simulink model "JX_Kinect_multi_sync"  (Simulink 7.7)
settings: Solver=ode4  StartTime=0.0  StopTime=inf  FixedStep=sample_time  RelTol=1e-3
InitFcn:
  | sample_time=0.005;%0.004;%0.0025;%0.02;
  | DeltaT = 0.02;
  | g = 9.81;
  | H0 = g%0.3165;
  | Kl = 1;
  | 
  | Omega_r = 1.6;%for Horizontal reference
  | Zeta_r = 1; %for Horizontal reference
  | Omega = 1.8;%for Horizontal Control
  | Zeta = 0.5;    %for Horizontal Control
  | 
  | Omega_h_r = 2.5; %for vertical reference
  | Zeta_h_r = 0.8;  %for vertical reference
  | Omega_h = 2.7;    %for vertical control
  | Zeta_h = 0.8;         %for vertical control
  | PI=pi;
  | 
  | Mass = 1.15;
  | Acc_Max = 4;
  | Acc_Max_h = 4;
  | 
  | Max_RP = 60;
  | 
  | % for NN
  | n = 5;
  | r = 3;
  | n2 = 5;
  | NN_ST = 0.02;
  | 
  | GAMA_V = 6;
  | gama_V_e = 0.01;
  | 
  | GAMA_W = GAMA_V;
  | gama_W_e =0.01;
  | 
  | % deadzone
  | NN_Deadzone_Z = 0;
  | 
  | % inputs nomalizaton parameters
  | NN_Z_y_min = -3;
  | NN_Z_y_max = 0.5;
  | 
  | NN_Z_v_max = 8;
  | NN_Z_v_min = -NN_Z_v_max;
  | 
  | % alpha = 0.034;
  | alpha = 1;
  | % c_f = 0.0015;
  | c_f = 0.001;
  | c_y_tilt = 1*0.5;
  | 
  | %for WK paras
  | Heightcontrol = 0.08;
  | Scale_Factor=1;
  | yoffset=0;
  | 
  | load MaoBi_Oct04_2_int.mat
  | MB_Interp.time = [];
undefined symbols (not defined in the file or in its folder): DiscIntNeverNeededParam
libraries: simulink x15, X330_Control x6, dspadpt3 x6, nid_lib x2
(part 1 of 4)
settings Model: Creator=ttcl3  LastModifiedBy=Jx
settings SolverCC: MaxConsecutiveMinStep=auto
settings DebuggingCC: MultiTaskRateTransMsg=warning
settings SFSimCC: SimParseCustomCode=off

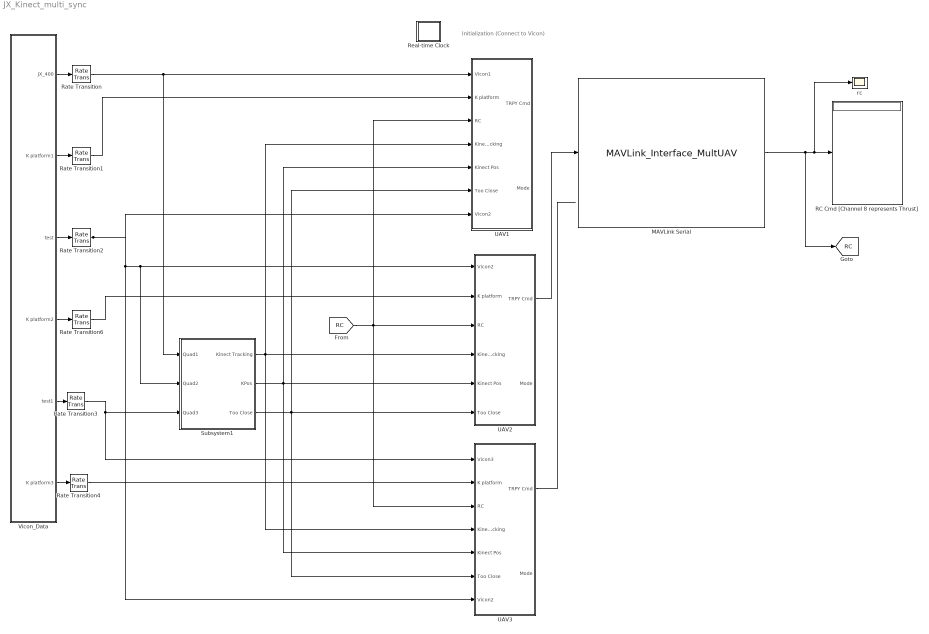
== system JX_Kinect_multi_sync ==
  note: Initialization
      | (Connect to Vicon)
  MAVLink Serial : S-Function  FunctionName=MAVLink_Interface_MultUAV  Parameters=COM_Port,Baud_Rate,MSG_INPUT,MSG_OUTPUT  EnableBusSupport=off  mask{COM_Port='COM6', Baud_Rate=57600, RC_SCALED=on, Quad_1=off, Quad_2=on, Quad_3=off}
      mask prompts: COM_Port "COM Port"; Baud_Rate "Baud Rate"; RC_SCALED "RC CHANNELS SCALED"; Quad_1 "Quad No 1"; Quad_2 "Quad No 2"; Quad_3 "Quad No 3"
      mask init:
      | MSG_ID_NUM_INPUT = [uint8(196) uint8(197) uint8(198)];
      | MSG_ID_NAME_INPUT = [Quad_1 Quad_2 Quad_3];
      | 
      | MSG_ID_NUM_OUTPUT = [uint8(34)];
      | MSG_ID_NAME_OUTPUT = [RC_SCALED];
      | 
      | idx_input = find(MSG_ID_NAME_INPUT);
      | MSG_INPUT = MSG_ID_NUM_INPUT(idx_input);
      | 
      | idx_output = find(MSG_ID_NAME_OUTPUT);
      | MSG_OUTPUT = MSG_ID_NUM_OUTPUT(idx_output);
      mask TabNameString: Setting,Setting,Output Message,Input Message,Input Message,Input Message
      mask Display:
      | % Block image
      | image(imread('10-inch Quad Heat Map.png'));
      | 
      | %Label block
      | fprintf('MAVLink Serial\n%s\n%dbps', COM_Port,  Baud_Rate)
      | 
      | 
      | %Label input ports
      | 
      | in = 1;
      | if (Quad_1 == 1)
      |     port_label('input', in, 'Quad 1');
      |     in = in + 1;
      | end
      | if (Quad_2 == 1)
      |     port_label('input', in, 'Quad 2');
      |     in = in + 1;
      | end
      | 
      | if (Quad_3 == 1)
      |     port_label('input', in, 'Quad 3');
      |     in = in + 1;
      | end
      | 
      | %Label output ports
      | 
      | out = 1;
      | if (RC_SCALED == 1)
      |     port_label('output', out, 'RC CMD');
      |     out = out + 1;
      | end
  RC Cmd [Channel 8 represents Thrust] : Display
  Rate Transition{,1..4,6} (6 alike) : RateTransition  OutPortSampleTime=0.02
  Real-time Clock : Subsystem  mask(Real-time Clock){sample_time=0.02, tolerance=1}
      mask prompts: sample_time "Synchronize with real-time every n seconds:"; tolerance "Real-time warning tolerance (seconds):"
      mask help: Real-time Synchronization Block
      mask Help: This block synchronizes simulation time with the PC real-time clock or UNIX system clock. The first dialog entry is the period at which the clock is checked to insure real-time synchronization. The second dialog entry is the number of seconds that the simulation time must be within real-time before a warning is printed.
      mask Display: plot(0,0,100,100,[40,60,60,54,54,64,69,76,82,77,81,83,83,81,78,74,70,64,57,49,41,35,32,30,30,31,34,40,47,47,40,40],[90,90,85,85,80,79,76,87,80,70,64,57,49,41,33,28,24,22,21,23,25,31,37,46,56,65,73,78,80,85,85,90],[69,53,53],[64,50,73])
  Subsystem1 : Subsystem
  UAV1 : Subsystem
  UAV2 : Subsystem
  UAV3 : Subsystem
  Vicon_Data : Subsystem
  rc : Scope
      settings: TimeRange=10  YMin=-1  YMax=0.1
  tag scope: RC=global
  wires:
  MAVLink Serial/1 -> [RC], RC Cmd [Channel 8 represents Thrust]/1, rc/1
  Vicon_Data/1(JX_400) -> Rate Transition/1
  Vicon_Data/2(K platform1) -> Rate Transition1/1
  Rate Transition/1 -> UAV1/1(Vicon1), Subsystem1/1(Quad1)
  Rate Transition1/1 -> UAV1/2(K platform)
  Vicon_Data/3(test) -> Rate Transition2/1
  Rate Transition2/1 -> UAV1/7(Vicon2), UAV3/7(Vicon2), UAV2/1(Vicon2), Subsystem1/2(Quad2)
  Vicon_Data/4(K platform2) -> Rate Transition6/1
  Vicon_Data/5(test1) -> Rate Transition3/1
  Rate Transition3/1 -> UAV3/1(Vicon3), Subsystem1/3(Quad3)
  UAV3/1(TRPY Cmd) -> ?
  Vicon_Data/6(K platform3) -> Rate Transition4/1
  Rate Transition4/1 -> UAV3/2(K platform)
  Rate Transition6/1 -> UAV2/2(K platform)
  [RC] -> UAV1/3(RC), UAV2/3(RC), UAV3/3(RC)
  Subsystem1/1(Kinect Tracking) -> UAV2/4(Kinect Tracking), UAV1/4(Kinect Tracking), UAV3/4(Kinect Tracking)
  Subsystem1/2(KPos) -> UAV2/5(Kinect Pos), UAV1/5(Kinect Pos), UAV3/5(Kinect Pos)
  Subsystem1/3(Too Close) -> UAV1/6(Too Close), UAV2/6(Too Close), UAV3/6(Too Close)
  UAV2/1(TRPY Cmd) -> MAVLink Serial/1

== system JX_Kinect_multi_sync/Real-time Clock ==
  Real-time Clock : S-Function  FunctionName=rtclock  Parameters=sample_time, tolerance  EnableBusSupport=off

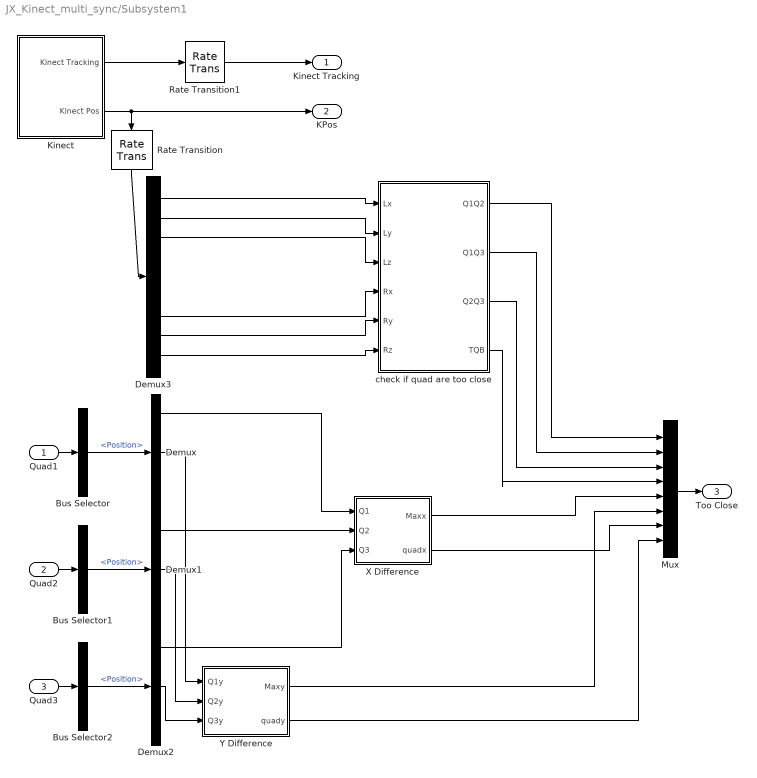
== system JX_Kinect_multi_sync/Subsystem1 ==
  Quad1 : Inport
  Quad2 : Inport  Port=2
  Quad3 : Inport  Port=3
  Bus Selector : BusSelector  OutputSignals=Position
  Bus Selector1 : BusSelector  OutputSignals=Position
  Bus Selector2 : BusSelector  OutputSignals=Position
  Demux : Demux  Outputs=3
  Demux1 : Demux  Outputs=3
  Demux2 : Demux  Outputs=3
  Demux3 : Demux  Outputs=9
  Kinect : Subsystem
  Mux : Mux  Inputs=8
  Rate Transition : RateTransition
  Rate Transition1 : RateTransition
  X Difference : Subsystem
  Y Difference : Subsystem
  check if quad are too close : Stateflow chart  TreatAsAtomicUnit=on
  Kinect Tracking : Outport
  KPos : Outport  Port=2
  Too Close : Outport  Port=3
  wires:
  Kinect/2(Kinect Pos) -> KPos/1, Rate Transition/1
  Kinect/1(Kinect Tracking) -> Rate Transition1/1
  Bus Selector/1 -> Demux/1  "<Position>"
  Bus Selector1/1 -> Demux1/1  "<Position>"
  Bus Selector2/1 -> Demux2/1  "<Position>"
  Quad2/1 -> Bus Selector1/1
  Quad3/1 -> Bus Selector2/1
  Quad1/1 -> Bus Selector/1
  Demux3/1 -> check if quad are too close/1(Lx)
  Demux3/2 -> check if quad are too close/2(Ly)
  Demux3/3 -> check if quad are too close/3(Lz)
  Demux3/7 -> check if quad are too close/4(Rx)
  Demux3/8 -> check if quad are too close/5(Ry)
  Demux3/9 -> check if quad are too close/6(Rz)
  Demux/1 -> X Difference/1(Q1)
  Demux/2 -> Y Difference/1(Q1y)
  Demux1/1 -> X Difference/2(Q2)
  Demux2/1 -> X Difference/3(Q3)
  check if quad are too close/1(Q1Q2) -> Mux/1
  check if quad are too close/2(Q1Q3) -> Mux/2
  check if quad are too close/3(Q2Q3) -> Mux/3
  Mux/1 -> Too Close/1
  check if quad are too close/4(TQB) -> Mux/4
  Y Difference/1(Maxy) -> Mux/6
  X Difference/1(Maxx) -> Mux/5
  X Difference/2(quadx) -> Mux/7
  Y Difference/2(quady) -> Mux/8
  Demux1/2 -> Y Difference/2(Q2y)
  Demux2/2 -> Y Difference/3(Q3y)
  Rate Transition/1 -> Demux3/1
  Rate Transition1/1 -> Kinect Tracking/1

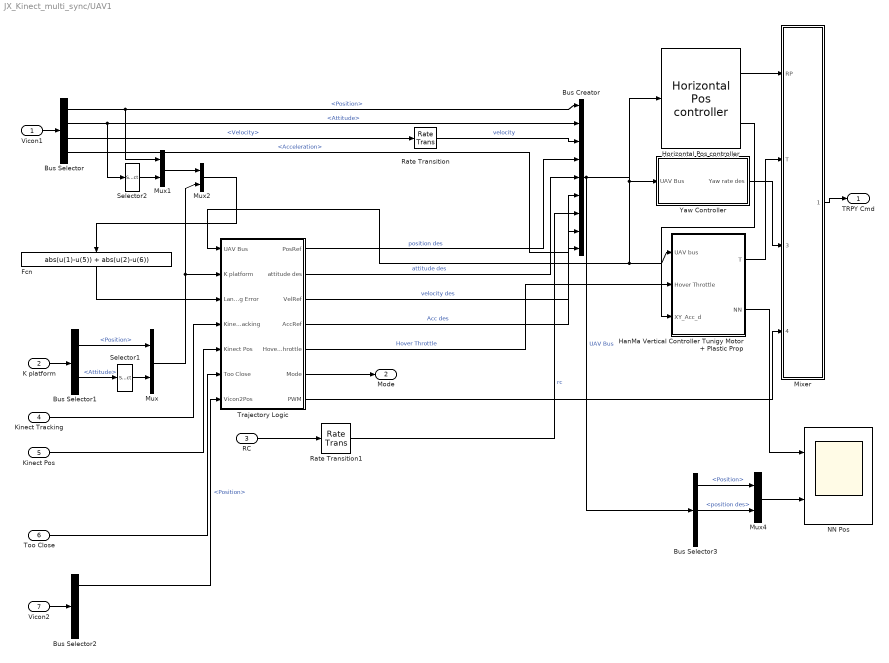
== system JX_Kinect_multi_sync/UAV1 ==
  Vicon1 : Inport
  K platform : Inport  Port=2
  RC : Inport  Port=3
  Kinect Tracking : Inport  Port=4
  Kinect Pos : Inport  Port=5
  Too Close : Inport  Port=6
  Vicon2 : Inport  Port=7
  Bus Creator : BusCreator  Inputs=9
  Bus Selector : BusSelector  OutputSignals=Position,Attitude,Velocity,Acceleration
  Bus Selector1 : BusSelector  OutputSignals=Position,Attitude
  Bus Selector2 : BusSelector  OutputSignals=Position,Attitude,Velocity,Acceleration
  Bus Selector3 : BusSelector  OutputSignals=Position,position des,Attitude
  Fcn : Fcn  Expr=abs(u(1)-u(5)) + abs(u(2)-u(6))
  HanMa Vertical Controller Tunigy Motor + Plastic Prop : Subsystem  mask{Omega_h=Omega_h, Zeta_h=Zeta_h, PID_I_h=0, mass=0.85}
      mask prompts: Omega_h "Omega (P Gain  = Omega^2)"; Zeta_h "Zeta (D Gain = 2*Omega*Zeta)"; PID_I_h "I Gain"
      mask TabNameString: Control Paramters,Control Paramters,Control Paramters,Mass
  Horizontal Pos controller : X330_Control/Horizontal Pos controller  SystemSampleTime=-1  Max_RP=Max_RP  Omega=Omega  PID_i=2  Zeta=Zeta
  Mixer : Subsystem
  Mux{,1..2,4} (4 alike) : Mux  Inputs=2
  NN Pos : Scope  NumInputPorts=2
      settings: TimeRange=90  YMin=-5~-2  YMax=10~2  SaveName=ScopeData3
  Rate Transition : RateTransition  OutPortSampleTime=0.02
  Rate Transition1 : RateTransition  OutPortSampleTime=0.02
  Selector1 : Selector  InputPortWidth=3  IndexOptions=Index vector (dialog)  Indices=[3]  OutputSizes=1
  Selector2 : Selector  InputPortWidth=3  IndexOptions=Index vector (dialog)  Indices=[3]  OutputSizes=1
  Trajectory Logic : Subsystem
  Yaw Controller : Subsystem
  TRPY Cmd : Outport
  Mode : Outport  Port=2
  wires:
  Horizontal Pos controller/1 -> Mixer/1(RP)
  Rate Transition/1 -> Bus Creator/3  "velocity"
  Rate Transition1/1 -> Bus Creator/7  "rc"
  Bus Creator/1 -> Yaw Controller/1(UAV Bus), Trajectory Logic/1(UAV Bus), HanMa Vertical Controller Tunigy Motor + Plastic Prop/1(UAV bus), Horizontal Pos controller/1, Bus Selector3/1  "UAV Bus"
  Yaw Controller/1(Yaw rate des) -> Mixer/3(Yaw rate)
  HanMa Vertical Controller Tunigy Motor + Plastic Prop/1(T) -> Mixer/2(T)
  Bus Selector/4 -> Bus Creator/8  "<Acceleration>"
  Trajectory Logic/1(PosRef) -> Bus Creator/4  "position des"
  Trajectory Logic/2(attitude des) -> Bus Creator/5  "attitude des"
  Trajectory Logic/3(VelRef) -> Bus Creator/6  "velocity des"
  Trajectory Logic/5(HoverThrottle) -> HanMa Vertical Controller Tunigy Motor + Plastic Prop/2(Hover Throttle)  "Hover Throttle"
  Bus Selector/1 -> Mux1/1, Bus Creator/1  "<Position>"
  Bus Selector/2 -> Selector2/1, Bus Creator/2  "<Attitude>"
  Bus Selector/3 -> Rate Transition/1  "<Velocity>"
  Vicon1/1 -> Bus Selector/1
  Mixer/1(XYZ RPY) -> TRPY Cmd/1
  Trajectory Logic/4(AccRef) -> Bus Creator/9  "Acc des"
  Mux/1 -> Mux2/2, Trajectory Logic/2(K platform)
  Trajectory Logic/6(Mode) -> Mode/1
  RC/1 -> Rate Transition1/1
  Trajectory Logic/7(PWM) -> Mixer/4(PWM)
  K platform/1 -> Bus Selector1/1
  Bus Selector1/1 -> Mux/1  "<Position>"
  Bus Selector1/2 -> Selector1/1  "<Attitude>"
  Selector1/1 -> Mux/2
  Selector2/1 -> Mux1/2
  Mux2/1 -> Fcn/1
  Mux1/1 -> Mux2/1
  Fcn/1 -> Trajectory Logic/3(Landing Error)
  Horizontal Pos controller/2 -> HanMa Vertical Controller Tunigy Motor + Plastic Prop/3(XY_Acc_d)
  Mux4/1 -> NN Pos/2
  Bus Selector3/1 -> Mux4/1  "<Position>"
  Bus Selector3/2 -> Mux4/2  "<position des>"
  HanMa Vertical Controller Tunigy Motor + Plastic Prop/2(NN) -> NN Pos/1
  Kinect Tracking/1 -> Trajectory Logic/4(Kinect Tracking)
  Kinect Pos/1 -> Trajectory Logic/5(Kinect Pos)
  Too Close/1 -> Trajectory Logic/6(Too Close)
  Vicon2/1 -> Bus Selector2/1
  Bus Selector2/1 -> Trajectory Logic/7(Vicon2Pos)  "<Position>"

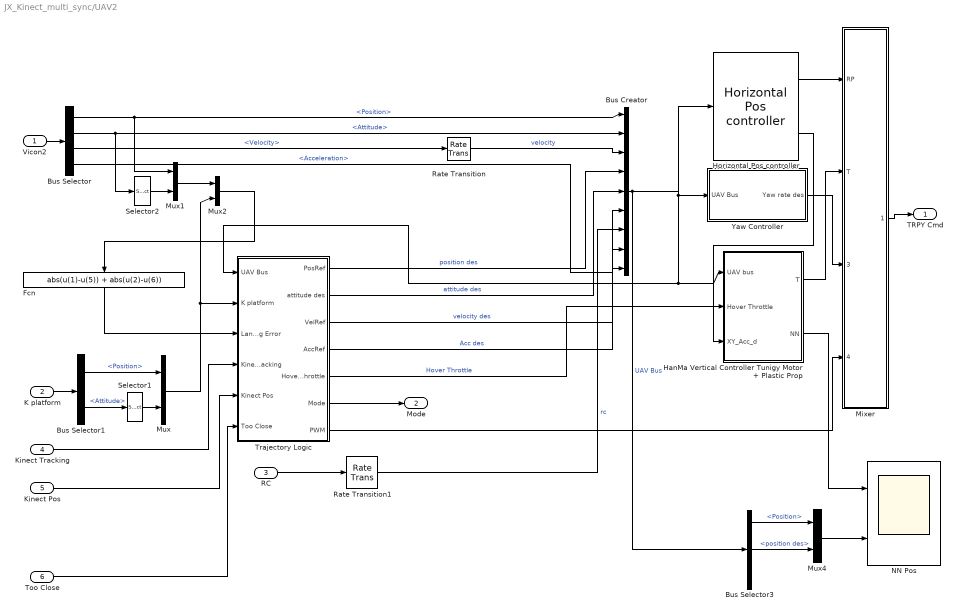
== system JX_Kinect_multi_sync/UAV2 ==
  Vicon2 : Inport
  K platform : Inport  Port=2
  RC : Inport  Port=3
  Kinect Tracking : Inport  Port=4
  Kinect Pos : Inport  Port=5
  Too Close : Inport  Port=6
  Bus Creator : BusCreator  Inputs=9
  Bus Selector : BusSelector  OutputSignals=Position,Attitude,Velocity,Acceleration
  Bus Selector1 : BusSelector  OutputSignals=Position,Attitude
  Bus Selector3 : BusSelector  OutputSignals=Position,position des,Attitude
  Fcn : Fcn  Expr=abs(u(1)-u(5)) + abs(u(2)-u(6))
  HanMa Vertical Controller Tunigy Motor + Plastic Prop : Subsystem  mask{Omega_h=Omega_h, Zeta_h=Zeta_h, PID_I_h=0, mass=0.85}
      mask prompts: Omega_h "Omega (P Gain  = Omega^2)"; Zeta_h "Zeta (D Gain = 2*Omega*Zeta)"; PID_I_h "I Gain"
      mask TabNameString: Control Paramters,Control Paramters,Control Paramters,Mass
  Horizontal Pos controller : X330_Control/Horizontal Pos controller  SystemSampleTime=-1  Max_RP=Max_RP  Omega=Omega  PID_i=2  Zeta=Zeta
  Mixer : Subsystem
  Mux{,1..2,4} (4 alike) : Mux  Inputs=2
  NN Pos : Scope  NumInputPorts=2
      settings: TimeRange=90  YMin=-5~-2  YMax=10~2  SaveName=ScopeData3
  Rate Transition : RateTransition  OutPortSampleTime=0.02
  Rate Transition1 : RateTransition  OutPortSampleTime=0.02
  Selector1 : Selector  InputPortWidth=3  IndexOptions=Index vector (dialog)  Indices=[3]  OutputSizes=1
  Selector2 : Selector  InputPortWidth=3  IndexOptions=Index vector (dialog)  Indices=[3]  OutputSizes=1
  Trajectory Logic : Subsystem
  Yaw Controller : Subsystem
  TRPY Cmd : Outport
  Mode : Outport  Port=2
  wires:
  Horizontal Pos controller/1 -> Mixer/1(RP)
  Rate Transition/1 -> Bus Creator/3  "velocity"
  Rate Transition1/1 -> Bus Creator/7  "rc"
  Bus Creator/1 -> Yaw Controller/1(UAV Bus), Trajectory Logic/1(UAV Bus), HanMa Vertical Controller Tunigy Motor + Plastic Prop/1(UAV bus), Horizontal Pos controller/1, Bus Selector3/1  "UAV Bus"
  Yaw Controller/1(Yaw rate des) -> Mixer/3(Yaw rate)
  HanMa Vertical Controller Tunigy Motor + Plastic Prop/1(T) -> Mixer/2(T)
  Bus Selector/4 -> Bus Creator/8  "<Acceleration>"
  Trajectory Logic/1(PosRef) -> Bus Creator/4  "position des"
  Trajectory Logic/2(attitude des) -> Bus Creator/5  "attitude des"
  Trajectory Logic/3(VelRef) -> Bus Creator/6  "velocity des"
  Trajectory Logic/5(HoverThrottle) -> HanMa Vertical Controller Tunigy Motor + Plastic Prop/2(Hover Throttle)  "Hover Throttle"
  Bus Selector/1 -> Mux1/1, Bus Creator/1  "<Position>"
  Bus Selector/2 -> Selector2/1, Bus Creator/2  "<Attitude>"
  Bus Selector/3 -> Rate Transition/1  "<Velocity>"
  Vicon2/1 -> Bus Selector/1
  Mixer/1(XYZ RPY) -> TRPY Cmd/1
  Trajectory Logic/4(AccRef) -> Bus Creator/9  "Acc des"
  Mux/1 -> Mux2/2, Trajectory Logic/2(K platform)
  Trajectory Logic/6(Mode) -> Mode/1
  RC/1 -> Rate Transition1/1
  Trajectory Logic/7(PWM) -> Mixer/4(PWM)
  K platform/1 -> Bus Selector1/1
  Bus Selector1/1 -> Mux/1  "<Position>"
  Bus Selector1/2 -> Selector1/1  "<Attitude>"
  Selector1/1 -> Mux/2
  Selector2/1 -> Mux1/2
  Mux2/1 -> Fcn/1
  Mux1/1 -> Mux2/1
  Fcn/1 -> Trajectory Logic/3(Landing Error)
  Horizontal Pos controller/2 -> HanMa Vertical Controller Tunigy Motor + Plastic Prop/3(XY_Acc_d)
  Mux4/1 -> NN Pos/2
  Bus Selector3/1 -> Mux4/1  "<Position>"
  Bus Selector3/2 -> Mux4/2  "<position des>"
  HanMa Vertical Controller Tunigy Motor + Plastic Prop/2(NN) -> NN Pos/1
  Kinect Tracking/1 -> Trajectory Logic/4(Kinect Tracking)
  Kinect Pos/1 -> Trajectory Logic/5(Kinect Pos)
  Too Close/1 -> Trajectory Logic/6(Too Close)

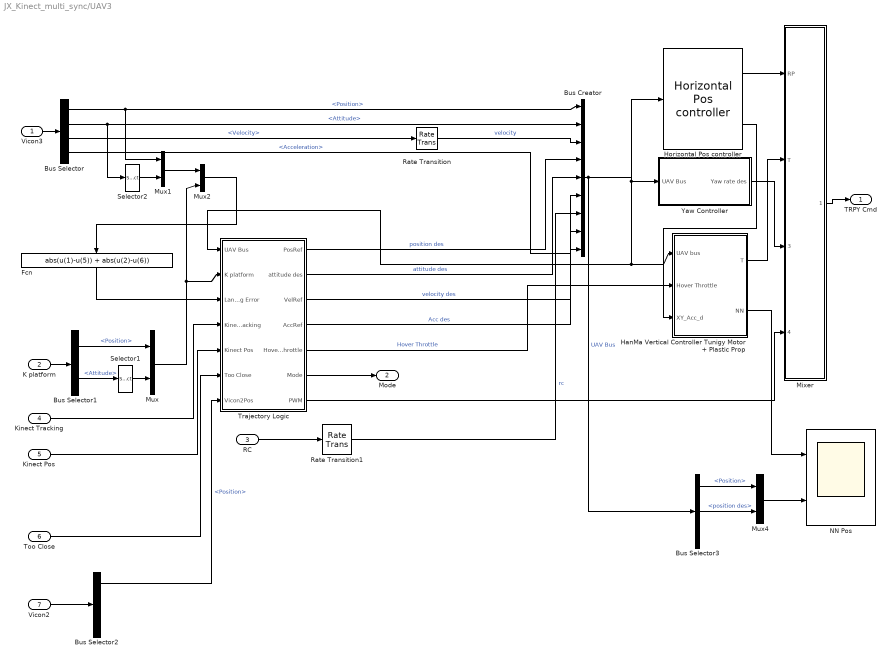
== system JX_Kinect_multi_sync/UAV3 ==
  Vicon3 : Inport
  K platform : Inport  Port=2
  RC : Inport  Port=3
  Kinect Tracking : Inport  Port=4
  Kinect Pos : Inport  Port=5
  Too Close : Inport  Port=6
  Vicon2 : Inport  Port=7
  Bus Creator : BusCreator  Inputs=9
  Bus Selector : BusSelector  OutputSignals=Position,Attitude,Velocity,Acceleration
  Bus Selector1 : BusSelector  OutputSignals=Position,Attitude
  Bus Selector2 : BusSelector  OutputSignals=Position,Attitude,Velocity,Acceleration
  Bus Selector3 : BusSelector  OutputSignals=Position,position des,Attitude
  Fcn : Fcn  Expr=abs(u(1)-u(5)) + abs(u(2)-u(6))
  HanMa Vertical Controller Tunigy Motor + Plastic Prop : Subsystem  mask{Omega_h=Omega_h, Zeta_h=Zeta_h, PID_I_h=0, mass=0.85}
      mask prompts: Omega_h "Omega (P Gain  = Omega^2)"; Zeta_h "Zeta (D Gain = 2*Omega*Zeta)"; PID_I_h "I Gain"
      mask TabNameString: Control Paramters,Control Paramters,Control Paramters,Mass
  Horizontal Pos controller : X330_Control/Horizontal Pos controller  SystemSampleTime=-1  Max_RP=Max_RP  Omega=Omega  PID_i=2  Zeta=Zeta
  Mixer : Subsystem
  Mux{,1..2,4} (4 alike) : Mux  Inputs=2
  NN Pos : Scope  NumInputPorts=2
      settings: TimeRange=90  YMin=-5~-2  YMax=10~2  SaveName=ScopeData3
  Rate Transition : RateTransition  OutPortSampleTime=0.02
  Rate Transition1 : RateTransition  OutPortSampleTime=0.02
  Selector1 : Selector  InputPortWidth=3  IndexOptions=Index vector (dialog)  Indices=[3]  OutputSizes=1
  Selector2 : Selector  InputPortWidth=3  IndexOptions=Index vector (dialog)  Indices=[3]  OutputSizes=1
  Trajectory Logic : Subsystem
  Yaw Controller : Subsystem
  TRPY Cmd : Outport
  Mode : Outport  Port=2
  wires:
  Horizontal Pos controller/1 -> Mixer/1(RP)
  Rate Transition/1 -> Bus Creator/3  "velocity"
  Rate Transition1/1 -> Bus Creator/7  "rc"
  Bus Creator/1 -> Yaw Controller/1(UAV Bus), Trajectory Logic/1(UAV Bus), HanMa Vertical Controller Tunigy Motor + Plastic Prop/1(UAV bus), Horizontal Pos controller/1, Bus Selector3/1  "UAV Bus"
  Yaw Controller/1(Yaw rate des) -> Mixer/3(Yaw rate)
  HanMa Vertical Controller Tunigy Motor + Plastic Prop/1(T) -> Mixer/2(T)
  Bus Selector/4 -> Bus Creator/8  "<Acceleration>"
  Trajectory Logic/1(PosRef) -> Bus Creator/4  "position des"
  Trajectory Logic/2(attitude des) -> Bus Creator/5  "attitude des"
  Trajectory Logic/3(VelRef) -> Bus Creator/6  "velocity des"
  Trajectory Logic/5(HoverThrottle) -> HanMa Vertical Controller Tunigy Motor + Plastic Prop/2(Hover Throttle)  "Hover Throttle"
  Bus Selector/1 -> Mux1/1, Bus Creator/1  "<Position>"
  Bus Selector/2 -> Selector2/1, Bus Creator/2  "<Attitude>"
  Bus Selector/3 -> Rate Transition/1  "<Velocity>"
  Vicon3/1 -> Bus Selector/1
  Mixer/1(XYZ RPY) -> TRPY Cmd/1
  Trajectory Logic/4(AccRef) -> Bus Creator/9  "Acc des"
  Mux/1 -> Mux2/2, Trajectory Logic/2(K platform)
  Trajectory Logic/6(Mode) -> Mode/1
  RC/1 -> Rate Transition1/1
  Trajectory Logic/7(PWM) -> Mixer/4(PWM)
  K platform/1 -> Bus Selector1/1
  Bus Selector1/1 -> Mux/1  "<Position>"
  Bus Selector1/2 -> Selector1/1  "<Attitude>"
  Selector1/1 -> Mux/2
  Selector2/1 -> Mux1/2
  Mux2/1 -> Fcn/1
  Mux1/1 -> Mux2/1
  Fcn/1 -> Trajectory Logic/3(Landing Error)
  Horizontal Pos controller/2 -> HanMa Vertical Controller Tunigy Motor + Plastic Prop/3(XY_Acc_d)
  Mux4/1 -> NN Pos/2
  Bus Selector3/1 -> Mux4/1  "<Position>"
  Bus Selector3/2 -> Mux4/2  "<position des>"
  HanMa Vertical Controller Tunigy Motor + Plastic Prop/2(NN) -> NN Pos/1
  Kinect Tracking/1 -> Trajectory Logic/4(Kinect Tracking)
  Kinect Pos/1 -> Trajectory Logic/5(Kinect Pos)
  Too Close/1 -> Trajectory Logic/6(Too Close)
  Vicon2/1 -> Bus Selector2/1
  Bus Selector2/1 -> Trajectory Logic/7(Vicon2Pos)  "<Position>"

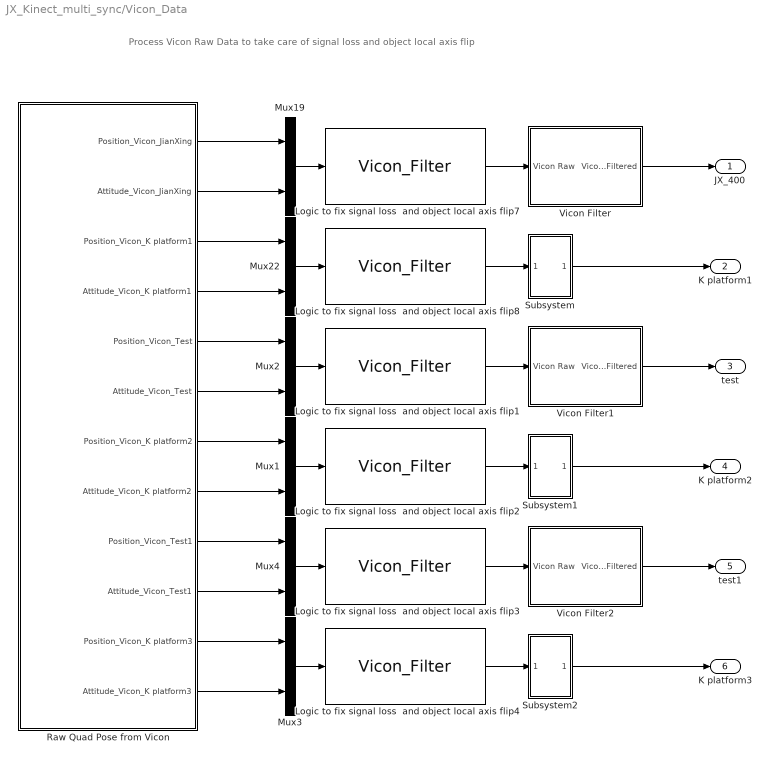
== system JX_Kinect_multi_sync/Vicon_Data ==
  note: Process Vicon Raw Data to take care of signal loss and object local axis flip
  Logic to fix signal loss  and object local axis flip{1..4,7..8} (6 alike) : M-S-Function  FunctionName=Vicon_Filter
  Mux{1..4,19,22} (6 alike) : Mux  Inputs=2
  Raw Quad Pose from Vicon : Subsystem
  Subsystem : Subsystem
  Subsystem1 : Subsystem
  Subsystem2 : Subsystem
  Vicon Filter : Subsystem
  Vicon Filter1 : Subsystem
  Vicon Filter2 : Subsystem
  JX_400 : Outport
  K platform1 : Outport  Port=2
  test : Outport  Port=3
  K platform2 : Outport  Port=4
  test1 : Outport  Port=5
  K platform3 : Outport  Port=6
  wires:
  Raw Quad Pose from Vicon/4(Attitude_Vicon_K platform1) -> Mux22/2
  Raw Quad Pose from Vicon/3(Position_Vicon_K platform1) -> Mux22/1
  Raw Quad Pose from Vicon/2(Attitude_Vicon_JianXing) -> Mux19/2
  Raw Quad Pose from Vicon/1(Position_Vicon_JianXing) -> Mux19/1
  Subsystem/1(Out1) -> K platform1/1
  Logic to fix signal loss  and object local axis flip8/1 -> Subsystem/1(In1)
  Mux22/1 -> Logic to fix signal loss  and object local axis flip8/1
  Vicon Filter/1(Vicon Filtered) -> JX_400/1
  Logic to fix signal loss  and object local axis flip7/1 -> Vicon Filter/1(Vicon Raw)
  Mux19/1 -> Logic to fix signal loss  and object local axis flip7/1
  Logic to fix signal loss  and object local axis flip1/1 -> Vicon Filter1/1(Vicon Raw)
  Vicon Filter1/1(Vicon Filtered) -> test/1
  Raw Quad Pose from Vicon/6(Attitude_Vicon_Test) -> Mux2/2
  Raw Quad Pose from Vicon/5(Position_Vicon_Test) -> Mux2/1
  Mux2/1 -> Logic to fix signal loss  and object local axis flip1/1
  Subsystem1/1(Out1) -> K platform2/1
  Logic to fix signal loss  and object local axis flip2/1 -> Subsystem1/1(In1)
  Mux1/1 -> Logic to fix signal loss  and object local axis flip2/1
  Raw Quad Pose from Vicon/7(Position_Vicon_K platform2) -> Mux1/1
  Raw Quad Pose from Vicon/8(Attitude_Vicon_K platform2) -> Mux1/2
  Logic to fix signal loss  and object local axis flip3/1 -> Vicon Filter2/1(Vicon Raw)
  Vicon Filter2/1(Vicon Filtered) -> test1/1
  Raw Quad Pose from Vicon/10(Attitude_Vicon_Test1) -> Mux4/2
  Raw Quad Pose from Vicon/9(Position_Vicon_Test1) -> Mux4/1
  Mux4/1 -> Logic to fix signal loss  and object local axis flip3/1
  Subsystem2/1(Out1) -> K platform3/1
  Logic to fix signal loss  and object local axis flip4/1 -> Subsystem2/1(In1)
  Mux3/1 -> Logic to fix signal loss  and object local axis flip4/1
  Raw Quad Pose from Vicon/11(Position_Vicon_K platform3) -> Mux3/1
  Raw Quad Pose from Vicon/12(Attitude_Vicon_K platform3) -> Mux3/2

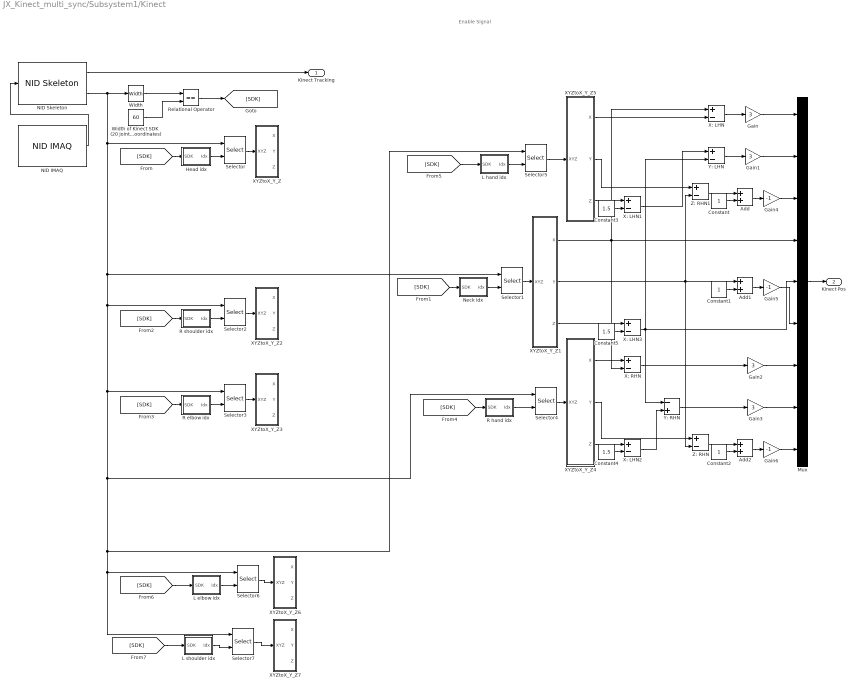
== system JX_Kinect_multi_sync/Subsystem1/Kinect ==
  note: Enable Signal
  Add : Sum
  Add1 : Sum
  Add2 : Sum
  Constant : Constant
  Constant1 : Constant
  Constant2 : Constant
  Constant3 : Constant  Value=1.5
  Constant4 : Constant  Value=1.5
  Constant5 : Constant  Value=1.5
  Gain{,1..3} (4 alike) : Gain  Gain=3
  Gain4 : Gain  Gain=-1
  Gain5 : Gain  Gain=-1
  Gain6 : Gain  Gain=-1
  Head idx : Subsystem
  L elbow idx : Subsystem
  L hand idx : Subsystem
  L shoulder idx : Subsystem
  Mux : Mux  Inputs=9
  NID IMAQ : nid_lib/NID IMAQ  imaq_depth=off  imaq_motion=off  imaq_image=off  view_point=off  imaq_skeleton=on  imaq_ir=off  mirror_image=off  imaq_sample_time=1/25  res_fps=VGA (640x480): 30 FPS  needPsiPose=off  angle_input=off  angle=0  angle_read=off  near_mode=off  seated_mode=off  skeleton_smooth=[0.5 0.5 0.5 0.05 0.04]  infer_skeleton=off
  NID Skeleton : nid_lib/NID Skeleton  num_of_skeleton_tracking=1  conv_XYZ_RW=on  viewer=off
  Neck idx : Subsystem
  R elbow idx : Subsystem
  R hand idx : Subsystem
  R shoulder idx : Subsystem
  Relational Operator : RelationalOperator  Operator===  OutDataTypeStr=boolean
  Selector{,1..7} (8 alike) : Selector  NumberOfDimensions=3  InputPortWidth=3  IndexOptions=Select all,Index vector (port),Select all  Indices=[1 3],1,1  OutputSizes=1,1,1
  Width : Width
  Width of Kinect SDK  (20 joints x 3 coordinates) : Constant  Value=60
  X: LHN{,1..3} (4 alike) : Sum  Inputs=+-
  X: RHN : Sum  Inputs=+-
  XYZtoX_Y_Z : Subsystem
  XYZtoX_Y_Z1 : Subsystem
  XYZtoX_Y_Z2 : Subsystem
  XYZtoX_Y_Z3 : Subsystem
  XYZtoX_Y_Z4 : Subsystem
  XYZtoX_Y_Z5 : Subsystem
  XYZtoX_Y_Z6 : Subsystem
  XYZtoX_Y_Z7 : Subsystem
  Y: LHN : Sum  Inputs=+-
  Y: RHN : Sum  Inputs=-+
  Z: RHN : Sum  Inputs=+-
  Z: RHN1 : Sum  Inputs=+-
  Kinect Tracking : Outport
  Kinect Pos : Outport  Port=2
  wires:
  Selector/1 -> XYZtoX_Y_Z/1(XYZ)
  Selector4/1 -> XYZtoX_Y_Z4/1(XYZ)
  Selector3/1 -> XYZtoX_Y_Z3/1(XYZ)
  Selector2/1 -> XYZtoX_Y_Z2/1(XYZ)
  [SDK] -> R hand idx/1(SDK)
  [SDK] -> R elbow idx/1(SDK)
  R elbow idx/1(Idx) -> Selector3/2
  [SDK] -> R shoulder idx/1(SDK)
  R shoulder idx/1(Idx) -> Selector2/2
  Selector1/1 -> XYZtoX_Y_Z1/1(XYZ)
  [SDK] -> Neck idx/1(SDK)
  Neck idx/1(Idx) -> Selector1/2
  NID Skeleton/1 -> Kinect Tracking/1
  [SDK] -> Head idx/1(SDK)
  Head idx/1(Idx) -> Selector/2
  Relational Operator/1 -> [SDK]
  NID Skeleton/2 -> Selector3/1, Selector4/1, Selector5/1, Selector6/1, Selector7/1, Selector2/1, Selector1/1, Selector/1, Width/1
  Width of Kinect SDK  (20 joints x 3 coordinates)/1 -> Relational Operator/2
  Width/1 -> Relational Operator/1
  NID IMAQ/1 -> NID Skeleton/1
  [SDK] -> L hand idx/1(SDK)
  [SDK] -> L elbow idx/1(SDK)
  [SDK] -> L shoulder idx/1(SDK)
  L hand idx/1(Idx) -> Selector5/2
  L elbow idx/1(Idx) -> Selector6/2
  L shoulder idx/1(Idx) -> Selector7/2
  Selector5/1 -> XYZtoX_Y_Z5/1(XYZ)
  Selector6/1 -> XYZtoX_Y_Z6/1(XYZ)
  Selector7/1 -> XYZtoX_Y_Z7/1(XYZ)
  R hand idx/1(Idx) -> Selector4/2
  XYZtoX_Y_Z5/1(X) -> X: LHN/2
  XYZtoX_Y_Z5/2(Y) -> Z: RHN1/1
  XYZtoX_Y_Z1/1(X) -> X: LHN/1, X: RHN/2, Mux/4
  XYZtoX_Y_Z1/2(Y) -> Z: RHN/2, Z: RHN1/2, Add1/1
  XYZtoX_Y_Z4/1(X) -> X: RHN/1
  XYZtoX_Y_Z4/2(Y) -> Z: RHN/1
  Z: RHN1/1 -> Add/1
  Constant/1 -> Add/2
  Constant1/1 -> Add1/2
  Z: RHN/1 -> Add2/1
  Constant2/1 -> Add2/2
  Mux/1 -> Kinect Pos/1
  Add1/1 -> Gain5/1
  Gain1/1 -> Mux/2
  Add/1 -> Gain4/1
  Y: LHN/1 -> Gain1/1
  X: LHN/1 -> Gain/1
  Gain3/1 -> Mux/8
  Add2/1 -> Gain6/1
  X: RHN/1 -> Gain2/1
  Y: RHN/1 -> Gain3/1
  Gain/1 -> Mux/1
  Gain2/1 -> Mux/7
  Gain4/1 -> Mux/3
  Gain5/1 -> Mux/6
  Gain6/1 -> Mux/9
  XYZtoX_Y_Z5/3(Z) -> X: LHN1/1
  Constant3/1 -> X: LHN1/2
  X: LHN1/1 -> Y: LHN/1
  XYZtoX_Y_Z4/3(Z) -> X: LHN2/1
  Constant4/1 -> X: LHN2/2
  X: LHN2/1 -> Y: RHN/2
  XYZtoX_Y_Z1/3(Z) -> X: LHN3/1
  Constant5/1 -> X: LHN3/2
  X: LHN3/1 -> Mux/5, Y: RHN/1, Y: LHN/2

== system JX_Kinect_multi_sync/Subsystem1/X Difference ==
  Q1 : Inport
  Q2 : Inport  Port=2
  Q3 : Inport  Port=3
  Abs : Abs
  Abs2 : Abs
  MATLAB Function : Stateflow chart  TreatAsAtomicUnit=on
  Subtract : Sum  Inputs=+-
  Subtract2 : Sum  Inputs=-+
  Maxx : Outport
  quadx : Outport  Port=2
  wires:
  Subtract2/1 -> Abs2/1
  Subtract/1 -> Abs/1
  Abs/1 -> MATLAB Function/1(x1)
  MATLAB Function/1(maxx) -> Maxx/1
  Q1/1 -> Subtract/1
  Q2/1 -> Subtract/2, Subtract2/1
  Q3/1 -> Subtract2/2
  Abs2/1 -> MATLAB Function/2(x2)
  MATLAB Function/2(Quad) -> quadx/1

== system JX_Kinect_multi_sync/Subsystem1/Y Difference ==
  Q1y : Inport
  Q2y : Inport  Port=2
  Q3y : Inport  Port=3
  MATLAB Function : Stateflow chart  TreatAsAtomicUnit=on
  Subtract : Sum  Inputs=-+
  Subtract2 : Sum  Inputs=+-
  Maxy : Outport
  quady : Outport  Port=2
  wires:
  Subtract2/1 -> MATLAB Function/1(y1)
  MATLAB Function/1(maxy) -> Maxy/1
  Subtract/1 -> MATLAB Function/2(y2)
  Q1y/1 -> Subtract2/1
  Q3y/1 -> Subtract/2
  Q2y/1 -> Subtract2/2, Subtract/1
  MATLAB Function/2(quady) -> quady/1

== system JX_Kinect_multi_sync/UAV1/HanMa Vertical Controller Tunigy Motor + Plastic Prop ==
  note: Manual Thrust
  UAV bus : Inport
  Hover Throttle : Inport  Port=2
  XY_Acc_d : Inport  Port=3
  Bus Selector : BusSelector  OutputSignals=Position,position des,rc,velocity,velocity des,Acc des
  Bus Selector3 : BusSelector  OutputSignals=rc
  Selector{1,3..5} (4 alike) : Selector  InputPortWidth=3  IndexOptions=Index vector (dialog)  Indices=[3]  OutputSizes=1
  Selector6 : Selector  InputPortWidth=4  IndexOptions=Index vector (dialog)  Indices=[3]  OutputSizes=1
  Selector7 : Selector  InputPortWidth=8  IndexOptions=Index vector (dialog)  Indices=[5]  OutputSizes=1
  Sum : Sum  Inputs=|-+
  Sum1 : Sum  Inputs=|-+
  Verticall Pos Controller : Subsystem
  T : Outport
  NN : Outport  Port=2
  wires:
  XY_Acc_d/1 -> Verticall Pos Controller/6(XY_Acc_d)
  Verticall Pos Controller/1("T  Commands [0, 1]") -> T/1  "T"
  Selector6/1 -> Verticall Pos Controller/5(Acc des)
  Bus Selector/6 -> Selector6/1  "<Acc des>"
  Hover Throttle/1 -> Verticall Pos Controller/4(Hover Throttle)
  Bus Selector/5 -> Selector5/1  "<velocity des>"
  Bus Selector/4 -> Selector3/1  "<velocity>"
  Selector5/1 -> Sum1/2
  Selector3/1 -> Sum1/1
  Sum1/1 -> Verticall Pos Controller/3(Vel Error), Verticall Pos Controller/10(Vel)  "Vel_error"
  Selector7/1 -> Verticall Pos Controller/2(Reset)  "reset"
  Bus Selector3/1 -> Selector7/1, Verticall Pos Controller/9(RC)  "<rc>"
  Selector1/1 -> Sum/2, Verticall Pos Controller/7(Height Ref)
  Selector4/1 -> Sum/1, Verticall Pos Controller/8(Height)
  Sum/1 -> Verticall Pos Controller/1(Pos Error)  "Down error"
  Bus Selector/2 -> Selector1/1  "<position des>"
  Bus Selector/1 -> Selector4/1  "<Position>"
  Bus Selector/3 -> Bus Selector3/1  "<rc>"
  UAV bus/1 -> Bus Selector/1
  Verticall Pos Controller/2(NN) -> NN/1

== system JX_Kinect_multi_sync/UAV1/Mixer ==
  note: 7x1 vector (usec, XYZRPY)
  RP : Inport
  T : Inport  Port=2
  Yaw rate : Inport  Port=3
  PWM : Inport  Port=4
  Gain : Gain  Gain=180/pi
  Manual Switch : simulink/Signal Routing/Manual Switch  SystemSampleTime=-1  sw=1  action=0  varsize=off
  Mux1 : Mux  Inputs=5
  PWM (1000-close; 2000-open) : Constant  Value=1600  SampleTime=0.02
  PWM (1000-close; 2000-open)1 : Constant  Value=1200  SampleTime=0.02
  "[-1, 1]" : Fcn  Expr=u(1)*2-1
  id : Constant  SampleTime=0.02
  XYZ RPY : Outport
  wires:
  Mux1/1 -> XYZ RPY/1
  T/1 -> "[-1, 1]"/1
  RP/1 -> Gain/1
  Yaw rate/1 -> Mux1/3
  id/1 -> Mux1/5
  PWM (1000-close; 2000-open)/1 -> Manual Switch/1
  PWM (1000-close; 2000-open)1/1 -> Manual Switch/2
  PWM/1 -> Mux1/4
  Gain/1 -> Mux1/2
  "[-1, 1]"/1 -> Mux1/1

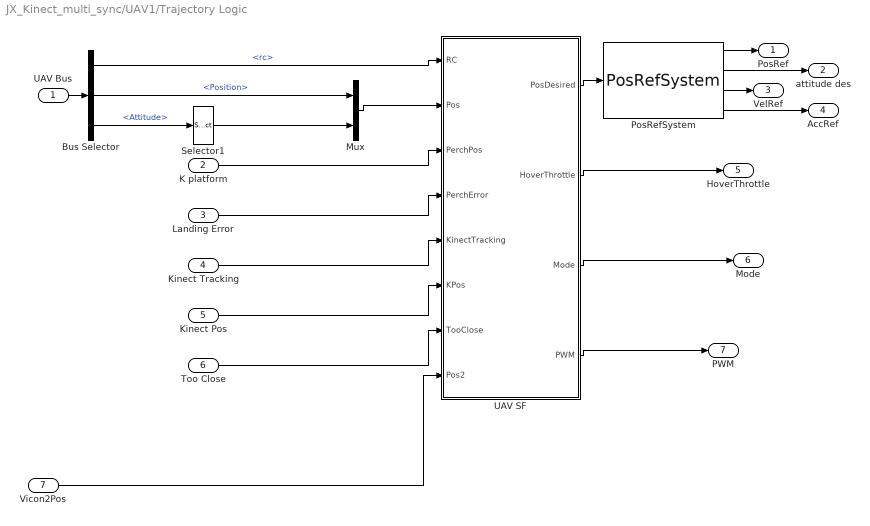
== system JX_Kinect_multi_sync/UAV1/Trajectory Logic ==
  UAV Bus : Inport
  K platform : Inport  Port=2
  Landing Error : Inport  Port=3
  Kinect Tracking : Inport  Port=4
  Kinect Pos : Inport  Port=5
  Too Close : Inport  Port=6
  Vicon2Pos : Inport  Port=7
  Bus Selector : BusSelector  OutputSignals=rc,Position,Attitude
  Mux : Mux  Inputs=2
  PosRefSystem : X330_Control/PosRefSystem  SystemSampleTime=-1  Omega_r=Omega_r  Zeta_r=Zeta_r  Acc_Max=Acc_Max  Omega_h_r=Omega_h_r  Zeta_h_r=Zeta_h_r  Acc_h_Max=Acc_Max_h
      link override Pos XY Lim: UpperLimit=2  LowerLimit=-2
  Selector1 : Selector  InputPortWidth=3  IndexOptions=Index vector (dialog)  Indices=[3]  OutputSizes=1
  UAV SF : Stateflow chart  TreatAsAtomicUnit=on
  PosRef : Outport
  attitude des : Outport  Port=2
  VelRef : Outport  Port=3
  AccRef : Outport  Port=4
  HoverThrottle : Outport  Port=5
  Mode : Outport  Port=6
  PWM : Outport  Port=7
  wires:
  UAV SF/1(PosDesired) -> PosRefSystem/1
  Bus Selector/1 -> UAV SF/1(RC)  "<rc>"
  UAV SF/2(HoverThrottle) -> HoverThrottle/1
  K platform/1 -> UAV SF/3(PerchPos)
  UAV SF/3(Mode) -> Mode/1
  UAV Bus/1 -> Bus Selector/1
  Bus Selector/2 -> Mux/1  "<Position>"
  Bus Selector/3 -> Selector1/1  "<Attitude>"
  Selector1/1 -> Mux/2
  Mux/1 -> UAV SF/2(Pos)
  UAV SF/4(PWM) -> PWM/1
  Landing Error/1 -> UAV SF/4(PerchError)
  PosRefSystem/1 -> PosRef/1
  PosRefSystem/3 -> VelRef/1
  PosRefSystem/4 -> AccRef/1
  PosRefSystem/2 -> attitude des/1
  Kinect Tracking/1 -> UAV SF/5(KinectTracking)
  Kinect Pos/1 -> UAV SF/6(KPos)
  Too Close/1 -> UAV SF/7(TooClose)
  Vicon2Pos/1 -> UAV SF/8(Pos2)

== system JX_Kinect_multi_sync/UAV1/Yaw Controller ==
  UAV Bus : Inport
  Bus Selector1 : BusSelector  OutputSignals=Attitude,attitude des,rc
  Gain : Gain  Gain=180/pi
  Heading : Subsystem  AncestorBlock=simulink/Continuous/PID Controller  DialogController=pidpack.PIDConfig.pidDDGCreate  DialogControllerArgs=DataTag0  mask(PID 1dof){Controller=PI, TimeDomain=Discrete-time, SampleTime=0.02, IntegratorMethod=Trapezoidal, FilterMethod=Trapezoidal, Form=Parallel, P=3, I=1, D=0, N=100, InitialConditionSource=internal, InitialConditionForIntegrator=0, InitialConditionForFilter=0, ExternalReset=rising, IgnoreLimit=off, ZeroCross=on, LimitOutput=on, UpperSaturationLimit=300*pi/180, LowerSaturationLimit=-300*pi/180, LinearizeAsGain=off, AntiWindupMode=none, Kb=1, TrackingMode=off, Kt=1, RndMeth=Floor, SaturateOnIntegerOverflow=off, LockScale=off, PParamMin=[], PParamMax=[], PParamDataTypeStr=Inherit: Inherit via internal rule, IParamMin=[], IParamMax=[], IParamDataTypeStr=Inherit: Inherit via internal rule, DParamMin=[], DParamMax=[], DParamDataTypeStr=Inherit: Inherit via internal rule, NParamMin=[], NParamMax=[], NParamDataTypeStr=Inherit: Inherit via internal rule, KbParamMin=[], KbParamMax=[], KbParamDataTypeStr=Inherit: Inherit via internal rule, KtParamMin=[], KtParamMax=[], KtParamDataTypeStr=Inherit: Inherit via internal rule, POutMin=[], POutMax=[], POutDataTypeStr=Inherit: Inherit via internal rule, IOutMin=[], IOutMax=[], IOutDataTypeStr=Inherit: Inherit via internal rule, DOutMin=[], DOutMax=[], DOutDataTypeStr=Inherit: Inherit via internal rule, NOutMin=[], NOutMax=[], NOutDataTypeStr=Inherit: Inherit via internal rule, KbOutMin=[], KbOutMax=[], KbOutDataTypeStr=Inherit: Inherit via internal rule, KtOutMin=[], KtOutMax=[], KtOutDataTypeStr=Inherit: Inherit via internal rule, IntegratorOutMin=[], IntegratorOutMax=[], IntegratorOutDataTypeStr=Inherit: Inherit via internal rule, FilterOutMin=[], FilterOutMax=[], FilterOutDataTypeStr=Inherit: Inherit via internal rule, SumOutMin=[], SumOutMax=[], SumOutDataTypeStr=Inherit: Inherit via internal rule, SumI1OutMin=[], SumI1OutMax=[], SumI1OutDataTypeStr=Inherit: Inherit via internal rule, SumI2OutMin=[], SumI2OutMax=[], SumI2OutDataTypeStr=Inherit: Inherit via internal rule, SumI3OutMin=[], SumI3OutMax=[], SumI3OutDataTypeStr=Inherit: Inherit via internal rule, SumDOutMin=[], SumDOutMax=[], SumDOutDataTypeStr=Inherit: Inherit via internal rule, SumAccumDataTypeStr=Inherit: Inherit via internal rule, SumI1AccumDataTypeStr=Inherit: Inherit via internal rule, SumI2AccumDataTypeStr=Inherit: Inherit via internal rule, SumI3AccumDataTypeStr=Inherit: Inherit via internal rule, SumDAccumDataTypeStr=Inherit: Inherit via internal rule, SaturationOutMin=[], SaturationOutMax=[], SaturationOutDataTypeStr=Inherit: Same as input, IntegratorContinuousStateAttributes='', IntegratorStateIdentifier=, IntegratorStateMustResolveToSignalObject=off, IntegratorRTWStateStorageClass=Auto, IntegratorRTWStateStorageTypeQualifier=, FilterContinuousStateAttributes='', FilterStateIdentifier=, FilterStateMustResolveToSignalObject=off, FilterRTWStateStorageClass=Auto, FilterRTWStateStorageTypeQualifier=}
      mask prompts: TimeDomain "Time domain:"; SampleTime "Sample time (-1 for inherited):"; IntegratorMethod "Integrator method:"; FilterMethod "Filter method:"; P "Proportional (P):"; I "Integral (I):"; D "Derivative (D):"; N "Filter coefficient (N):"; InitialConditionSource "Source:"; InitialConditionForIntegrator "Integrator:"; InitialConditionForFilter "Filter:"; ExternalReset "External reset:"; IgnoreLimit "Ignore reset when linearizing"; ZeroCross "Enable zero-crossing detection"; LimitOutput "Limit output"; UpperSaturationLimit "Upper saturation limit:"; LowerSaturationLimit "Lower saturation limit:"; LinearizeAsGain "Ignore saturation when linearizing"; AntiWindupMode "Anti-windup method:"; Kb "Back-calculation coefficient (Kb):"; TrackingMode "Enable tracking mode"; Kt "Tracking coefficient (Kt):"; RndMeth "Integer rounding mode:"; SaturateOnIntegerOverflow "Saturate on integer overflow"; LockScale "Lock data type settings against changes by the fixed-point tools"; PParamMin "P parameter minimum:"; PParamMax "P parameter maximum:"; PParamDataTypeStr "P parameter:"; IParamMin "I parameter minimum:"; IParamMax "I parameter maximum:"; IParamDataTypeStr "I parameter:"; DParamMin "D parameter minimum:"; DParamMax "D parameter maximum:"; DParamDataTypeStr "D parameter:"; NParamMin "N parameter minimum:"; NParamMax "N parameter maximum:"; NParamDataTypeStr "N parameter:"; KbParamMin "Kb parameter minimum:"; KbParamMax "Kb parameter maximum:"; KbParamDataTypeStr "Kb parameter:"; KtParamMin "Kt parameter minimum:"; KtParamMax "Kt parameter maximum:"; KtParamDataTypeStr "Kt parameter:"; POutMin "P product output minimum:"; POutMax "P product output maximum:"; POutDataTypeStr "P product output:"; IOutMin "I product output minimum:"; IOutMax "I product output maximum:"; IOutDataTypeStr "I product output:"; DOutMin "D product output minimum:"; DOutMax "D product output maximum:"; DOutDataTypeStr "D product output:"; NOutMin "N product output minimum:"; NOutMax "N product output maximum:"; NOutDataTypeStr "N product output:"; KbOutMin "Kb product output minimum:"; KbOutMax "Kb product output maximum:"; KbOutDataTypeStr "Kb product output:"; KtOutMin "Kt product output minimum:"; KtOutMax "Kt product output maximum:"; KtOutDataTypeStr "Kt product output:"; IntegratorOutMin "Integrator output minimum:"; IntegratorOutMax "Integrator output maximum:"; IntegratorOutDataTypeStr "Integrator output:"; FilterOutMin "Filter output minimum:"; FilterOutMax "Filter output maximum:"; FilterOutDataTypeStr "Filter output:"; SumOutMin "Sum output minimum:"; SumOutMax "Sum output maximum:"; SumOutDataTypeStr "Sum output:"; SumI1OutMin "SumI1 output minimum:"; SumI1OutMax "SumI1 output maximum:"; SumI1OutDataTypeStr "SumI1 output:"; SumI2OutMin "SumI2 output minimum:"; SumI2OutMax "SumI2 output maximum:"; SumI2OutDataTypeStr "SumI2 output:"; SumI3OutMin "SumI3 output minimum:"; SumI3OutMax "SumI3 output maximum:"; SumI3OutDataTypeStr "SumI3 output:"; SumDOutMin "SumD output minimum:"; SumDOutMax "SumD output maximum:"; SumDOutDataTypeStr "SumD output:"; SumAccumDataTypeStr "Accumulator of Sum:"; SumI1AccumDataTypeStr "Accumulator of SumI1:"; SumI2AccumDataTypeStr "Accumulator of SumI2:"; SumI3AccumDataTypeStr "Accumulator of SumI3:"; SumDAccumDataTypeStr "Accumulator of SumD:"; SaturationOutMin "Saturation output minimum:"; SaturationOutMax "Saturation output maximum:"; SaturationOutDataTypeStr "Saturation output:"; IntegratorContinuousStateAttributes "State name: (e.g., 'position')"; IntegratorStateIdentifier "State name:"; IntegratorStateMustResolveToSignalObject "State name must resolve to Simulink signal object"; IntegratorRTWStateStorageClass "Code generation storage class:"; IntegratorRTWStateStorageTypeQualifier "Code generation storage type qualifier:"; FilterContinuousStateAttributes "State name: (e.g., 'position')"; FilterStateIdentifier "State name:"; FilterStateMustResolveToSignalObject "State name must resolve to Simulink signal object"; FilterRTWStateStorageClass "Code generation storage class:"; FilterRTWStateStorageTypeQualifier "Code generation storage type qualifier:"
      mask help: This block implements continuous- and discrete-time PID control algorithms and includes advanced features such as anti-windup, external reset, and signal tracking. You can tune the PID gains automatically using the 'Tune...' button (requires Simulink Control Design).
      mask init:
      | pidpack.PIDConfig.configPID(gcbh);
      settings: DeleteFcn=pidpack.PIDConfig.closeTuner(gcbh)  ModelCloseFcn=pidpack.PIDConfig.closeTuner(gcbh)  NameChangeFcn=pidpack.PIDConfig.updateTunerName(gcbh)
      mask StyleString: popup(PID|PI|PD|P|I),popup(Continuous-time|Discrete-time),edit,popup(Forward Euler|Backward Euler|Trapezoidal),popup(Forward Euler|Backward Euler|Trapezoidal),popup(Ideal|Parallel),edit,edit,edit,edit,popup(internal|external),edit,edit,popup(none|rising|falling|either|level),checkbox,checkbox,checkbox,edit,edit,checkbox,popup(none|back-calculation|clamping),edit,checkbox,edit,popup(Ceiling|Convergent|Floor|Nearest|Round|Simplest|Zero),checkbox,checkbox,min,max,unidt({a=30|28|29|}{i=Inherit: Inherit via internal rule|Inherit: Same as input}{b=double|single|int8|uint8|int16|uint16|int32|uint32}{s=UDTBinaryPointMode|UDTSlopeBiasMode|UDTBestPrecisionMode}{g=UDTSignedSign|UDTUnsignedSign}),min,max,unidt({a=33|31|32|}{i=Inherit: Inherit via internal rule|Inherit: Same as input}{b=double|single|int8|uint8|int16|uint16|int32|uint32}{s=UDTBinaryPointMode|UDTSlopeBiasMode|UDTBestPrecisionMode}{g=UDTSignedSign|UDTUnsignedSign}),min,max,unidt({a=36|34|35|}{i=Inherit: Inherit via internal rule|Inherit: Same as input}{b=double|single|int8|uint8|int16|uint16|int32|uint32}{s=UDTBinaryPointMode|UDTSlopeBiasMode|UDTBestPrecisionMode}{g=UDTSignedSign|UDTUnsignedSign}),min,max,unidt({a=39|37|38|}{i=Inherit: Inherit via internal rule|Inherit: Same as input}{b=double|single|int8|uint8|int16|uint16|int32|uint32}{s=UDTBinaryPointMode|UDTSlopeBiasMode|UDTBestPrecisionMode}{g=UDTSignedSign|UDTUnsignedSign}),min,max,unidt({a=42|40|41|}{i=Inherit: Inherit via internal rule|Inherit: Same as input}{b=double|single|int8|uint8|int16|uint16|int32|uint32}{s=UDTBinaryPointMode|UDTSlopeBiasMode|UDTBestPrecisionMode}{g=UDTSignedSign|UDTUnsignedSign}),min,max,unidt({a=45|43|44|}{i=Inherit: Inherit via internal rule|Inherit: Same as input}{b=double|single|int8|uint8|int16|uint16|int32|uint32}{s=UDTBinaryPointMode|UDTSlopeBiasMode|UDTBestPrecisionMode}{g=UDTSignedSign|UDTUnsignedSign}),min,max,unidt({a=48|46|47|}{i=Inherit: Inherit via internal rule|Inherit: Inherit via back propagation|Inherit: Same as input}{b=double|single|int8|uint8|int16|uint16|int32|uint32}{s=UDTBinaryPointMode|UDTSlopeBiasMode}{g=UDTSignedSign|UDTUnsignedSign}),min,max,unidt({a=51|49|50|}{i=Inherit: Inherit via internal rule|Inherit: Inherit via back propagation|Inherit: Same as input}{b=double|single|int8|uint8|int16|uint16|int32|uint32}{s=UDTBinaryPointMode|UDTSlopeBiasMode}{g=UDTSignedSign|UDTUnsignedSign}),min,max,unidt({a=54|52|53|}{i=Inherit: Inherit via internal rule|Inherit: Inherit via back propagation|Inherit: Same as input}{b=double|single|int8|uint8|int16|uint16|int32|uint32}{s=UDTBinaryPointMode|UDTSlopeBiasMode}{g=UDTSignedSign|UDTUnsignedSign}),min,max,unidt({a=57|55|56|}{i=Inherit: Inherit via internal rule|Inherit: Inherit via back propagation|Inherit: Same as input}{b=double|single|int8|uint8|int16|uint16|int32|uint32}{s=UDTBinaryPointMode|UDTSlopeBiasMode}{g=UDTSignedSign|UDTUnsignedSign}),min,max,unidt({a=60|58|59|}{i=Inherit: Inherit via internal rule|Inherit: Inherit via back propagation|Inherit: Same as input}{b=double|single|int8|uint8|int16|uint16|int32|uint32}{s=UDTBinaryPointMode|UDTSlopeBiasMode}{g=UDTSignedSign|UDTUnsignedSign}),min,max,unidt({a=63|61|62|}{i=Inherit: Inherit via internal rule|Inherit: Inherit via back propagation|Inherit: Same as input}{b=double|single|int8|uint8|int16|uint16|int32|uint32}{s=UDTBinaryPointMode|UDTSlopeBiasMode}{g=UDTSignedSign|UDTUnsignedSign}),min,max,unidt({a=66|64|65|}{i=Inherit: Inherit via internal rule|Inherit: Inherit via back propagation}{b=double|single|int8|uint8|int16|uint16|int32|uint32}{s=UDTBinaryPointMode|UDTSlopeBiasMode}{g=UDTSignedSign|UDTUnsignedSign}),min,max,unidt({a=69|67|68|}{i=Inherit: Inherit via internal rule|Inherit: Inherit via back propagation}{b=double|single|int8|uint8|int16|uint16|int32|uint32}{s=UDTBinaryPointMode|UDTSlopeBiasMode}{g=UDTSignedSign|UDTUnsignedSign}),min,max,unidt({a=72|70|71|}{i=Inherit: Inherit via internal rule|Inherit: Inherit via back propagation|Inherit: Same as first input|Inherit: Same as accumulator}{b=double|single|int8|uint8|int16|uint16|int32|uint32}{s=UDTBinaryPointMode|UDTSlopeBiasMode}{g=UDTSignedSign|UDTUnsignedSign}),min,max,unidt({a=75|73|74|}{i=Inherit: Inherit via internal rule|Inherit: Inherit via back propagation|Inherit: Same as first input|Inherit: Same as accumulator}{b=double|single|int8|uint8|int16|uint16|int32|uint32}{s=UDTBinaryPointMode|UDTSlopeBiasMode}{g=UDTSignedSign|UDTUnsignedSign}),min,max,unidt({a=78|76|77|}{i=Inherit: Inherit via internal rule|Inherit: Inherit via back propagation|Inherit: Same as first input|Inherit: Same as accumulator}{b=double|single|int8|uint8|int16|uint16|int32|uint32}{s=UDTBinaryPointMode|UDTSlopeBiasMode}{g=UDTSignedSign|UDTUnsignedSign}),min,max,unidt({a=81|79|80|}{i=Inherit: Inherit via internal rule|Inherit: Inherit via back propagation|Inherit: Same as first input|Inherit: Same as accumulator}{b=double|single|int8|uint8|int16|uint16|int32|uint32}{s=UDTBinaryPointMode|UDTSlopeBiasMode}{g=UDTSignedSign|UDTUnsignedSign}),min,max,unidt({a=84|82|83|}{i=Inherit: Inherit via internal rule|Inherit: Inherit via back propagation|Inherit: Same as first input|Inherit: Same as accumulator}{b=double|single|int8|uint8|int16|uint16|int32|uint32}{s=UDTBinaryPointMode|UDTSlopeBiasMode}{g=UDTSignedSign|UDTUnsignedSign}),unidt({a=85|||}{i=Inherit: Inherit via internal rule|Inherit: Same as first input}{b=double|single|int8|uint8|int16|uint16|int32|uint32}{s=UDTBinaryPointMode|UDTSlopeBiasMode}{g=UDTSignedSign|UDTUnsignedSign}),unidt({a=86|||}{i=Inherit: Inherit via internal rule|Inherit: Same as first input}{b=double|single|int8|uint8|int16|uint16|int32|uint32}{s=UDTBinaryPointMode|UDTSlopeBiasMode}{g=UDTSignedSign|UDTUnsignedSign}),unidt({a=87|||}{i=Inherit: Inherit via internal rule|Inherit: Same as first input}{b=double|single|int8|uint8|int16|uint16|int32|uint32}{s=UDTBinaryPointMode|UDTSlopeBiasMode}{g=UDTSignedSign|UDTUnsignedSign}),unidt({a=88|||}{i=Inherit: Inherit via internal rule|Inherit: Same as first input}{b=double|single|int8|uint8|int16|uint16|int32|uint32}{s=UDTBinaryPointMode|UDTSlopeBiasMode}{g=UDTSignedSign|UDTUnsignedSign}),unidt({a=89|||}{i=Inherit: Inherit via internal rule|Inherit: Same as first input}{b=double|single|int8|uint8|int16|uint16|int32|uint32}{s=UDTBinaryPointMode|UDTSlopeBiasMode}{g=UDTSignedSign|UDTUnsignedSign}),min,max,unidt({a=92|90|91|}{i=Inherit: Inherit via back propagation|Inherit: Same as input}{b=double|single|int8|uint8|int16|uint16|int32|uint32}{s=UDTBinaryPointMode|UDTSlopeBiasMode}{g=UDTSignedSign|UDTUnsignedSign}),edit,edit,checkbox,popup(Auto|ExportedGlobal|ImportedExtern|ImportedExternPointer),edit,edit,edit,checkbox,popup(Auto|ExportedGlobal|ImportedExtern|ImportedExternPointer),edit
      mask Display:
      | disp('PI(z)')
      | port_label('input',1, '');
      | port_label('output',1, '');plot([0 4 4 7]+2,[0 0 8 8]+8);
      | plot([1 4 6]+2,[3 6 3]+8);
      | plot([0 4 6 10]+32,[0 0 8 8]+18);
  MATLAB Function : Stateflow chart  TreatAsAtomicUnit=on
  Selector5 : Selector  InputPortWidth=3  IndexOptions=Index vector (dialog)  Indices=[3]  OutputSizes=1
  Selector6 : Selector  InputPortWidth=3  IndexOptions=Index vector (dialog)  Indices=[3]  OutputSizes=1
  Selector7 : Selector  InputPortWidth=8  IndexOptions=Index vector (dialog)  Indices=[5]  OutputSizes=1
  Sum1 : Sum  Inputs=|-+
  Yaw rate des : Outport
  wires:
  Gain/1 -> Yaw rate des/1
  Selector5/1 -> Sum1/1
  Selector7/1 -> Heading/2(RESET)  "reset"
  Heading/1(y) -> Gain/1  "desire yaw rate"
  Bus Selector1/1 -> Selector5/1  "<Attitude>"
  UAV Bus/1 -> Bus Selector1/1
  MATLAB Function/1(y) -> Heading/1(u)
  Sum1/1 -> MATLAB Function/1(u)
  Selector6/1 -> Sum1/2
  Bus Selector1/2 -> Selector6/1  "<attitude des>"
  Bus Selector1/3 -> Selector7/1  "<rc>"

== system JX_Kinect_multi_sync/UAV2/HanMa Vertical Controller Tunigy Motor + Plastic Prop ==
  note: Manual Thrust
  UAV bus : Inport
  Hover Throttle : Inport  Port=2
  XY_Acc_d : Inport  Port=3
  Bus Selector : BusSelector  OutputSignals=Position,position des,rc,velocity,velocity des,Acc des
  Bus Selector3 : BusSelector  OutputSignals=rc
  Selector{1,3..5} (4 alike) : Selector  InputPortWidth=3  IndexOptions=Index vector (dialog)  Indices=[3]  OutputSizes=1
  Selector6 : Selector  InputPortWidth=4  IndexOptions=Index vector (dialog)  Indices=[3]  OutputSizes=1
  Selector7 : Selector  InputPortWidth=8  IndexOptions=Index vector (dialog)  Indices=[5]  OutputSizes=1
  Sum : Sum  Inputs=|-+
  Sum1 : Sum  Inputs=|-+
  Verticall Pos Controller : Subsystem
  T : Outport
  NN : Outport  Port=2
  wires:
  XY_Acc_d/1 -> Verticall Pos Controller/6(XY_Acc_d)
  Verticall Pos Controller/1("T  Commands [0, 1]") -> T/1  "T"
  Selector6/1 -> Verticall Pos Controller/5(Acc des)
  Bus Selector/6 -> Selector6/1  "<Acc des>"
  Hover Throttle/1 -> Verticall Pos Controller/4(Hover Throttle)
  Bus Selector/5 -> Selector5/1  "<velocity des>"
  Bus Selector/4 -> Selector3/1  "<velocity>"
  Selector5/1 -> Sum1/2
  Selector3/1 -> Sum1/1
  Sum1/1 -> Verticall Pos Controller/3(Vel Error), Verticall Pos Controller/10(Vel)  "Vel_error"
  Selector7/1 -> Verticall Pos Controller/2(Reset)  "reset"
  Bus Selector3/1 -> Selector7/1, Verticall Pos Controller/9(RC)  "<rc>"
  Selector1/1 -> Sum/2, Verticall Pos Controller/7(Height Ref)
  Selector4/1 -> Sum/1, Verticall Pos Controller/8(Height)
  Sum/1 -> Verticall Pos Controller/1(Pos Error)  "Down error"
  Bus Selector/2 -> Selector1/1  "<position des>"
  Bus Selector/1 -> Selector4/1  "<Position>"
  Bus Selector/3 -> Bus Selector3/1  "<rc>"
  UAV bus/1 -> Bus Selector/1
  Verticall Pos Controller/2(NN) -> NN/1

== system JX_Kinect_multi_sync/UAV2/Mixer ==
  note: 7x1 vector (usec, XYZRPY)
  RP : Inport
  T : Inport  Port=2
  Yaw rate : Inport  Port=3
  PWM : Inport  Port=4
  Gain : Gain  Gain=180/pi
  Manual Switch : simulink/Signal Routing/Manual Switch  SystemSampleTime=-1  sw=1  action=0  varsize=off
  Mux1 : Mux  Inputs=5
  PWM (1000-close; 2000-open) : Constant  Value=1600  SampleTime=0.02
  PWM (1000-close; 2000-open)1 : Constant  Value=1200  SampleTime=0.02
  "[-1, 1]" : Fcn  Expr=u(1)*2-1
  id : Constant  Value=2  SampleTime=0.02
  XYZ RPY : Outport
  wires:
  Mux1/1 -> XYZ RPY/1
  T/1 -> "[-1, 1]"/1
  RP/1 -> Gain/1
  Yaw rate/1 -> Mux1/3
  id/1 -> Mux1/5
  PWM (1000-close; 2000-open)/1 -> Manual Switch/1
  PWM (1000-close; 2000-open)1/1 -> Manual Switch/2
  PWM/1 -> Mux1/4
  Gain/1 -> Mux1/2
  "[-1, 1]"/1 -> Mux1/1
